simulink model "FPEC_sim"  (R2022b)
settings: Solver=VariableStepAuto  StartTime=0.0  StopTime=sim_time  RelTol=1e-3
values from neighbouring files (symbols this model uses):
  dco_white_free = 3e-5    (= 3e-05)    [convmat_fpec.m]    (also in convmat_lptv.m)
  dsm_white_free = 1/12    (= 0.0833333333333)    [convmat_fpec.m]    (also in convmat_lptv.m)
  fdco = fref*N    (= 630000000)    [convmat_fpec.m]    (also in convmat_lptv.m = 560000000)
  fdsm = fref*N/M    (= 157500000)    [convmat_fpec.m]    (also in convmat_lptv.m = 140000000)
  fref = 35e6    (= 35000000)    [convmat_fpec.m]    (also in convmat_lptv.m)
  Ki = Kp0/32    (= 0.0125)    [convmat_fpec.m]    (also in convmat_lptv.m)
  Kp = Kp0*N/P    (= 3.6)    [convmat_fpec.m]    (also in convmat_lptv.m = 0.4)
  Kpd = 300    [convmat_fpec.m]    (also in convmat_lptv.m)
  M = 4    [convmat_fpec.m]    (also in convmat_lptv.m)
  N = 18    [convmat_fpec.m]    (also in convmat_lptv.m = 16)
  noise_dco_en = 1    [convmat_fpec.m]    (also in convmat_lptv.m)
  noise_dsm_en = 1    [convmat_fpec.m]    (also in convmat_lptv.m)
  noise_ref_en = 1    [convmat_fpec.m]    (also in convmat_lptv.m)
  P = 2    [convmat_fpec.m]    (also in convmat_lptv.m = 16)
  tdc_white_free = 1/12/Kpd^2    (= 9.25925925926e-07)    [convmat_fpec.m]    (also in convmat_lptv.m)
libraries: simulink x3
settings Model: Creator=frank  LastModifiedBy=frank

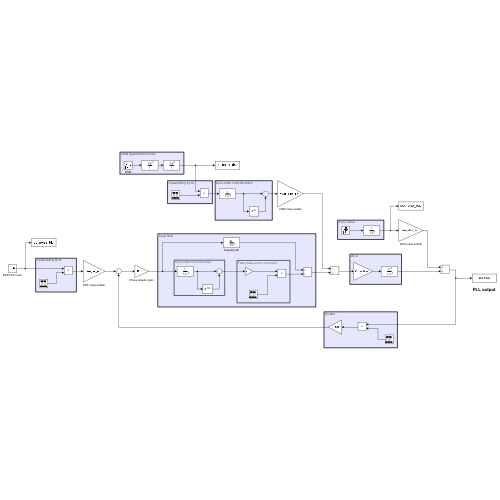
[thumbnail: Simulink's stored preview of the top-level diagram]
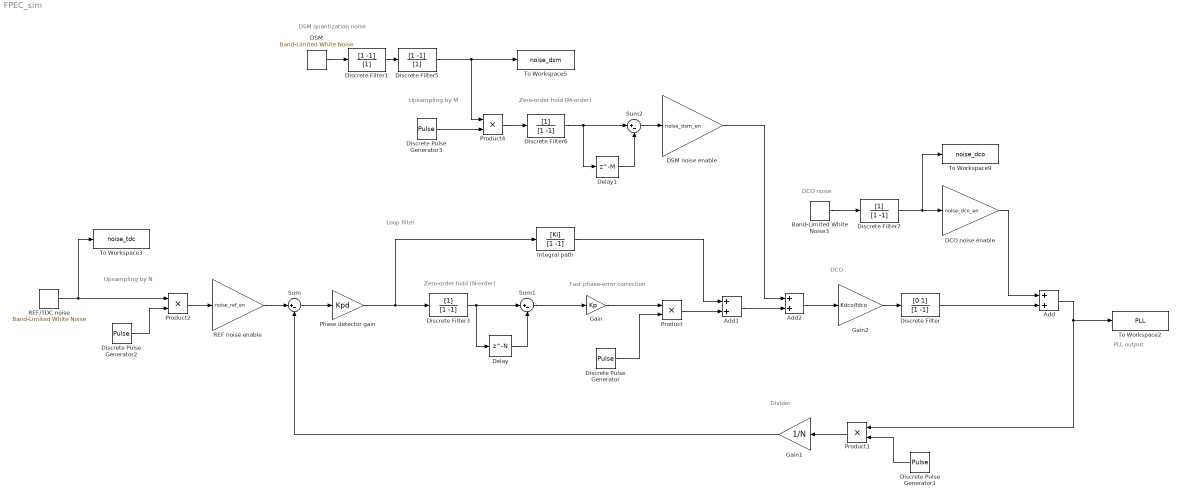
== system FPEC_sim ==
  note: DCO noise
  note: DCO
  note: Loop filter
  note: Divider
  note: Fast phase-error correction
  note: Zero-order hold (N-order)
  note: Upsampling by N
  note: Zero-order hold (M-order)
  note: Upsampling by M
  note: DSM quantization noise
  note: PLL output
  Add : Sum
  Add1 : Sum
  Add2 : Sum
  Band-Limited White Noise3 : simulink/Sources/Band-Limited White Noise  Cov=[dco_white_free/fdco]  Ts=1/fdco  seed=[446]
  DCO noise enable : Gain  Gain=noise_dco_en
  DSM : simulink/Sources/Band-Limited White Noise  Cov=[dsm_white_free/fdsm]  Ts=1/fdsm  seed=[357]
  DSM noise enable : Gain  Gain=noise_dsm_en
  Delay : Delay  DelayLength=N  InitialCondition=0
  Delay1 : Delay  DelayLength=M  InitialCondition=0
  Discrete Pulse Generator : DiscretePulseGenerator  Period=N  PulseWidth=P  SampleTime=1/fdco
  Discrete Pulse Generator1 : DiscretePulseGenerator  Period=N  SampleTime=1/fdco
  Discrete Pulse Generator2 : DiscretePulseGenerator  Period=N  SampleTime=1/fdco
  Discrete Pulse Generator3 : DiscretePulseGenerator  Period=M  SampleTime=1/fdco
  Discrete Filter : DiscreteFilter  Numerator=[0 1]  Denominator=[1 -1]
  Discrete Filter1 : DiscreteFilter  Numerator=[1 -1]  Denominator=[1]
  Discrete Filter3 : DiscreteFilter  Denominator=[1 -1]
  Discrete Filter5 : DiscreteFilter  Numerator=[1 -1]  Denominator=[1]
  Discrete Filter6 : DiscreteFilter  Denominator=[1 -1]
  Discrete Filter7 : DiscreteFilter  Denominator=[1 -1]
  Gain : Gain  Gain=Kp
  Gain1 : Gain  Gain=1/N
  Gain2 : Gain  Gain=Kdco/fdco
  Integral path : DiscreteFilter  Numerator=[Ki]  Denominator=[1 -1]
  Phase detector gain : Gain  Gain=Kpd
  Product{,1..2,4} (4 alike) : Product
  REF noise enable : Gain  Gain=noise_ref_en
  REF/TDC noise : simulink/Sources/Band-Limited White Noise  Cov=[tdc_white_free/fref]  Ts=1/fref  seed=[486]
  Sum : Sum  Inputs=|+-
  Sum1 : Sum  Inputs=|+-
  Sum2 : Sum  Inputs=|+-
  To Workspace2 : ToWorkspace  VariableName=PLL  SampleTime=-1
  To Workspace3 : ToWorkspace  VariableName=noise_tdc  SampleTime=-1
  To Workspace5 : ToWorkspace  VariableName=noise_dsm  SampleTime=-1
  To Workspace9 : ToWorkspace  VariableName=noise_dco  SampleTime=-1
  wires:
  Discrete Filter/1 -> Add/2
  Gain/1 -> Product/1
  Discrete Pulse Generator/1 -> Product/2
  Product/1 -> Add1/2
  Integral path/1 -> Add1/1
  Phase detector gain/1 -> Discrete Filter3/1, Integral path/1
  Sum/1 -> Phase detector gain/1
  Add/1 -> To Workspace2/1, Product1/1
  Discrete Pulse Generator1/1 -> Product1/2
  Gain2/1 -> Discrete Filter/1
  Discrete Filter3/1 -> Delay/1, Sum1/1
  Sum1/1 -> Gain/1
  Delay/1 -> Sum1/2
  Discrete Pulse Generator2/1 -> Product2/2
  Add2/1 -> Gain2/1
  Add1/1 -> Add2/2
  DSM/1 -> Discrete Filter1/1
  Discrete Filter1/1 -> Discrete Filter5/1
  Delay1/1 -> Sum2/2
  Discrete Filter5/1 -> To Workspace5/1, Product4/1
  Discrete Filter6/1 -> Delay1/1, Sum2/1
  Product4/1 -> Discrete Filter6/1
  Discrete Pulse Generator3/1 -> Product4/2
  Band-Limited White Noise3/1 -> Discrete Filter7/1
  REF/TDC noise/1 -> Product2/1, To Workspace3/1
  REF noise enable/1 -> Sum/1
  Product2/1 -> REF noise enable/1
  Sum2/1 -> DSM noise enable/1
  DSM noise enable/1 -> Add2/1
  Discrete Filter7/1 -> To Workspace9/1, DCO noise enable/1
  DCO noise enable/1 -> Add/1
  Product1/1 -> Gain1/1
  Gain1/1 -> Sum/2
